simulink model "DIL"  (R2025a)
settings: Solver=VariableStepAuto  StartTime=0.0  StopTime=10.0  RelTol=1e-3
settings Model: Creator=TAK  LastModifiedBy=TAK

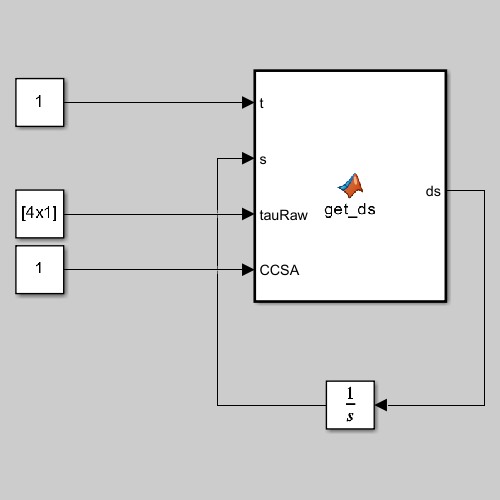
[thumbnail: Simulink's stored preview of the top-level diagram]
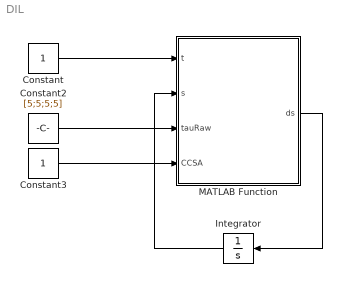
== system DIL ==
  Constant : Constant
  Constant2 : Constant  Value=[5;5;5;5]
  Constant3 : Constant
  Integrator : Integrator
  MATLAB Function : MATLAB Function  TreatAsAtomicUnit=on
  wires:
  Constant3/1 -> MATLAB Function/4(CCSA)
  Constant2/1 -> MATLAB Function/3(tauRaw)
  MATLAB Function/1(ds) -> Integrator/1
  Integrator/1 -> MATLAB Function/2(s)
  Constant/1 -> MATLAB Function/1(t)

== matlab function DIL/MATLAB Function ==
  data: ds output; t input; s input; tauRaw input; CCSA input; varCAR_struct parameter
function ds = get_ds(t, s, tauRaw, CCSA, varCAR_struct)
    ds = vehicle_ds(t, s, tauRaw, CCSA, varCAR_struct);
end
